simulink model "ProjectSimulink"  (R2023b)
settings: Solver=VariableStepAuto  StartTime=0.0  StopTime=10.0  RelTol=1e-3
libraries: simulink_extras x3
settings Model: Creator=pedro  LastModifiedBy=pedro

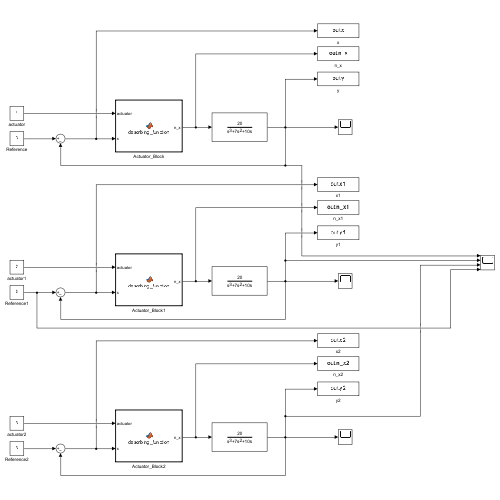
[thumbnail: Simulink's stored preview of the top-level diagram]
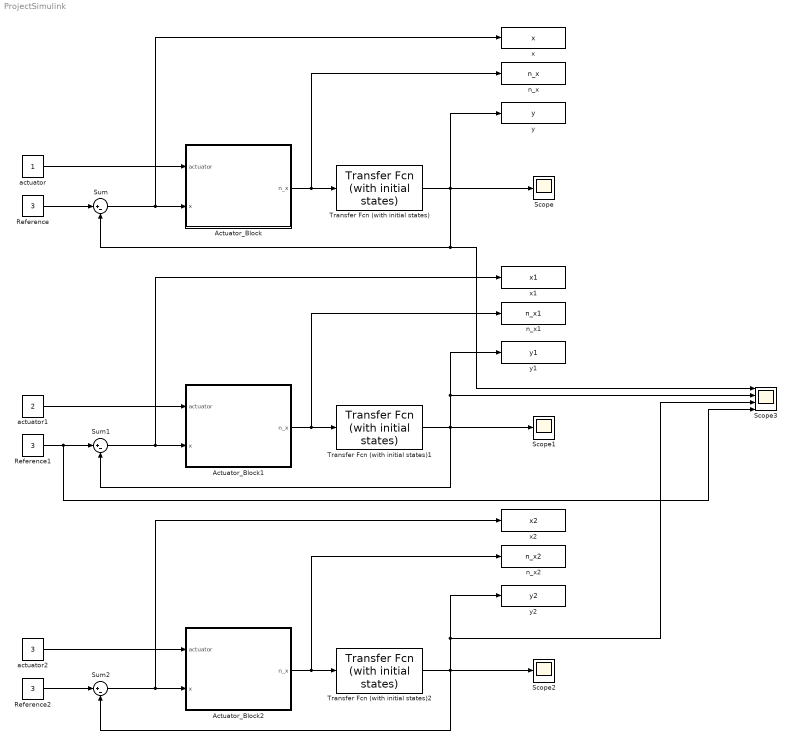
== system ProjectSimulink ==
  Actuator_Block : MATLAB Function  TreatAsAtomicUnit=on
  Actuator_Block1 : MATLAB Function  TreatAsAtomicUnit=on
  Actuator_Block2 : MATLAB Function  TreatAsAtomicUnit=on
  Reference : Constant  Value=3
  Reference1 : Constant  Value=3
  Reference2 : Constant  Value=3
  Scope : Scope
  Scope1 : Scope
  Scope2 : Scope
  Scope3 : Scope  NumInputPorts=4
  Sum : Sum  Inputs=|+-
  Sum1 : Sum  Inputs=|+-
  Sum2 : Sum  Inputs=|+-
  Transfer Fcn (with initial states) : simulink_extras/Additional Linear/Transfer Fcn (with initial states)  N=[20]  D="[1  7  10  0]"  X0=0
  Transfer Fcn (with initial states)1 : simulink_extras/Additional Linear/Transfer Fcn (with initial states)  N=[20]  D="[1  7  10  0]"  X0=0
  Transfer Fcn (with initial states)2 : simulink_extras/Additional Linear/Transfer Fcn (with initial states)  N=[20]  D="[1  7  10  0]"  X0=0
  actuator : Constant
  actuator1 : Constant  Value=2
  actuator2 : Constant  Value=3
  n_x : ToWorkspace  VariableName=n_x  SaveFormat=Timeseries  SampleTime=-1
  n_x1 : ToWorkspace  VariableName=n_x1  SaveFormat=Timeseries  SampleTime=-1
  n_x2 : ToWorkspace  VariableName=n_x2  SaveFormat=Timeseries  SampleTime=-1
  x : ToWorkspace  VariableName=x  SaveFormat=Timeseries  SampleTime=-1
  x1 : ToWorkspace  VariableName=x1  SaveFormat=Timeseries  SampleTime=-1
  x2 : ToWorkspace  VariableName=x2  SaveFormat=Timeseries  SampleTime=-1
  y : ToWorkspace  VariableName=y  SaveFormat=Timeseries  SampleTime=-1
  y1 : ToWorkspace  VariableName=y1  SaveFormat=Timeseries  SampleTime=-1
  y2 : ToWorkspace  VariableName=y2  SaveFormat=Timeseries  SampleTime=-1
  wires:
  Transfer Fcn (with initial states)/1 -> Sum/2, Scope3/1, Scope/1, y/1
  Sum/1 -> x/1, Actuator_Block/2(x)
  actuator/1 -> Actuator_Block/1(actuator)
  Actuator_Block/1(n_x) -> Transfer Fcn (with initial states)/1, n_x/1
  Reference/1 -> Sum/1
  Reference1/1 -> Scope3/4, Sum1/1
  Actuator_Block1/1(n_x) -> Transfer Fcn (with initial states)1/1, n_x1/1
  Transfer Fcn (with initial states)1/1 -> y1/1, Scope3/2, Sum1/2, Scope1/1
  actuator1/1 -> Actuator_Block1/1(actuator)
  Sum1/1 -> x1/1, Actuator_Block1/2(x)
  Reference2/1 -> Sum2/1
  Actuator_Block2/1(n_x) -> Transfer Fcn (with initial states)2/1, n_x2/1
  Transfer Fcn (with initial states)2/1 -> Scope3/3, y2/1, Sum2/2, Scope2/1
  actuator2/1 -> Actuator_Block2/1(actuator)
  Sum2/1 -> x2/1, Actuator_Block2/2(x)

== matlab function ProjectSimulink/Actuator_Block ==
  data: actuator input; x input; n_x output
function n_x = describing_function(actuator, x)

A = real(x);

if actuator == 1
    if A > 0
        N_A = 2-(4/pi)*(asin(complex(1/(2*A))) + (1/(2*A))*sqrt(complex(1-1/(4*A^2))));
    else
        N_A = -2-(4/pi)*(asin(complex(1/(2*A))) + (1/(2*A))*sqrt(complex(1-1/(4*A^2))));        
    end

elseif actuator == 2
    N_A = 4/(pi*A)*sqrt(complex(1-1/A^2));

else
    N_A = 2/(pi*A)*exp(-1i*asin(complex(2/A)));
end

n_x = real(N_A);

== matlab function ProjectSimulink/Actuator_Block2 ==
  data: actuator input; x input; n_x output
function n_x = describing_function(actuator, x)

A = real(x);

if actuator == 1
    if A > 0
        N_A = 2-(4/pi)*(asin(complex(1/(2*A))) + (1/(2*A))*sqrt(complex(1-1/(4*A^2))));
    else
        N_A = -2-(4/pi)*(asin(complex(1/(2*A))) + (1/(2*A))*sqrt(complex(1-1/(4*A^2))));        
    end

elseif actuator == 2
    N_A = 4/(pi*A)*sqrt(complex(1-1/A^2));

else
    N_A = 2/(pi*A)*exp(-1i*asin(complex(2/A)));
end

n_x = real(N_A);

== matlab function ProjectSimulink/Actuator_Block1 ==
  data: actuator input; x input; n_x output
function n_x = describing_function(actuator, x)

A = real(x);

if actuator == 1
    if A > 0
        N_A = 2-(4/pi)*(asin(complex(1/(2*A))) + (1/(2*A))*sqrt(complex(1-1/(4*A^2))));
    else
        N_A = -2-(4/pi)*(asin(complex(1/(2*A))) + (1/(2*A))*sqrt(complex(1-1/(4*A^2))));        
    end

elseif actuator == 2
    N_A = 4/(pi*A)*sqrt(complex(1-1/A^2));

else
    N_A = 2/(pi*A)*exp(-1i*asin(complex(2/A)));
end

n_x = real(N_A);
